simulink model "pendcartsim_nitin"  (R2021a)
settings: Solver=VariableStepAuto  StartTime=0.0  StopTime=100  RelTol=1e-3
values from neighbouring files (symbols this model uses):
  A = [0,1,0,0;0,-b/M,m*g/M,0;0,0,0,1;0,-b/M/l,g*(m+M)/M/l,0]    [sim_pendcart_nitin.m]
  B = [0;1/M;0;1/M/l]    [sim_pendcart_nitin.m]
  K = lqr(A,B,Q,R)    [sim_pendcart_nitin.m]
settings Model: Creator=MYPC  LastModifiedBy=MYPC
settings DataIOCC: ExternalInput=[xf]  InitialState=x0

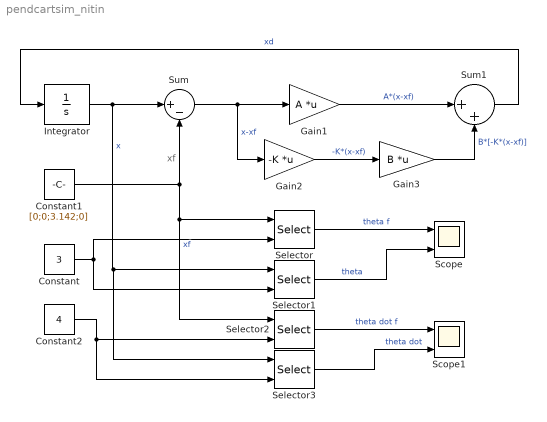
== system pendcartsim_nitin ==
  note: xf
  Constant : Constant  Value=3
  Constant1 : Constant  Value=[0;0;3.142;0]
  Constant2 : Constant  Value=4
  Gain1 : Gain  Gain=A  Multiplication=Matrix(K*u) (u vector)
  Gain2 : Gain  Gain=-K  Multiplication=Matrix(K*u) (u vector)
  Gain3 : Gain  Gain=B  Multiplication=Matrix(K*u) (u vector)
  Integrator : Integrator
  Scope : Scope  NumInputPorts=2
  Scope1 : Scope  NumInputPorts=2
  Selector{,1..3} (4 alike) : Selector  InputPortWidth=4  IndexOptions=Index vector (port)  Indices=[1 3]  OutputSizes=1
  Sum : Sum  Inputs=|+-
  Sum1 : Sum  Inputs=|++
  wires:
  Integrator/1 -> Selector3/1, Selector1/1, Sum/1  "x"
  Sum/1 -> Gain2/1, Gain1/1  "x-xf"
  Gain2/1 -> Gain3/1  "-K*(x-xf)"
  Gain3/1 -> Sum1/2  "B*[-K*(x-xf)]"
  Gain1/1 -> Sum1/1  "A*(x-xf)"
  Sum1/1 -> Integrator/1  "xd"
  Constant1/1 -> Selector2/1, Selector/1, Sum/2  "xf"
  Constant/1 -> Selector/2, Selector1/2
  Selector/1 -> Scope/1  "theta f"
  Selector1/1 -> Scope/2  "theta"
  Constant2/1 -> Selector3/2, Selector2/2
  Selector2/1 -> Scope1/1  "theta dot f"
  Selector3/1 -> Scope1/2  "theta dot"
